simulink model "purePursuitUSCity"  (R2022b)
settings: Solver=VariableStepAuto  StartTime=0.0  StopTime=Ts  RelTol=1e-3
PreLoadFcn:
  | setUpPurePursuitUSCity
model workspace (MAT data in the model file):
  firstWarning = 0
  originalScenarioChecksum = 'F73A6DA3C723D3CA73A6F931B7A52A9C'
values from neighbouring files (symbols this model uses):
  diffcurve = []    [setUpPurePursuitUSCity.m]
  L = data.ActorSpecifications.Length    [setUpPurePursuitUSCity.m]
  ld = 5    [setUpPurePursuitUSCity.m]
  psi_o = refPose(1,3)    [setUpPurePursuitUSCity.m]
  s = size(xRef)    [setUpPurePursuitUSCity.m]
  X_o = refPose(1,1)    [setUpPurePursuitUSCity.m]
  xRef = refPose(:,1)    [setUpPurePursuitUSCity.m]
  Y_o = -refPose(1,2)    [setUpPurePursuitUSCity.m]
  yRef = -refPose(:,2)    [setUpPurePursuitUSCity.m]
undefined symbols (not defined in the file or in its folder): data, deg, rad
libraries: autolibutils x4, autolibshared x3, vehdynlibviscommon x1, aerolibconvert2 x1, simulink_extras x1, drivingscenarioandsensors x1, robotalgslib x1, simulink x1, sim3dlib x1, vdynlib x1
(part 3 of 3)

== system purePursuitUSCity/Powertrain & Driveline/Driveline/FWD ==
  TPowertrain : Inport
  FWD : Gain  Gain=[1;1;0;0]
  TAxles : Outport  VectorParamsAs1DForOutWhenUnconnected=off
  wires:
  FWD/1 -> TAxles/1
  TPowertrain/1 -> FWD/1

== system purePursuitUSCity/Powertrain & Driveline/Driveline/RWD ==
  TPowertrain : Inport
  RWD : Gain  Gain=[0;0;1;1]
  TAxles : Outport  VectorParamsAs1DForOutWhenUnconnected=off
  wires:
  TPowertrain/1 -> RWD/1
  RWD/1 -> TAxles/1

== matlab function purePursuitUSCity/Final Trajectory Bird's-Eye Visualization/MATLAB Function ==
  data: pos input; egoActor output Bus: BusActorsActors; vel input; yaw input; yawRate input
function egoActor = packEgo(pos,vel,yaw,yawRate)
% Pack ego information into a single ego actor bus
%
% Imoprtant note:
% Output is a bus of type BusActorsActors. This is the same bus used by the
% Scenario Reader to output an individual actor. If you change the
% output bus name of Scenario Reader, change the output bus name here
% as well by clicking on 'Edit Data' in the menu above.

egoActor = struct(...
    'ActorID',67,...
    'Position', [pos(1) pos(2) 0], ...
    'Velocity', [vel(1) vel(2) 0], ...
    'Roll', 0, ...
    'Pitch', 0, ...
    'Yaw', yaw, ...
    'AngularVelocity', [0 0 yawRate]);

== matlab function purePursuitUSCity/Optimal Vel/MATLAB Function ==
  data: diffcurve input; y output; speed input; cx input; cy input; refX input; refY input; j output; j input
function [y,j]= fcn(diffcurve,speed,cx,cy,refX,refY,j)

dx = refX- x;
dy = [refY- y];
d= hypot(dx, dy);
[~, ind] = min(d);


if(j==floor(ind/10)) 
    
    if diffcurve(j)>0 && diffcurve(j)<0.5
        %vel(end+1)=30;
        speed=30;
        
    data.ActorSpecifications.Speed=speed;
    y=data.ActorSpecifications.Speed;
    
    elseif diffcurve(j)>=0.5 && diffcurve(j)<1
        %vel(end+1)=20;
        speed=20;
        
    data.ActorSpecifications.Speed=speed;
    y=data.ActorSpecifications.Speed;
    
    elseif diffcurve(j)>=1 && diffcurve(j)<1.5
        %vel(end+1)=10;
        speed=10;
    
    data.ActorSpecifications.Speed=speed;
    y=data.ActorSpecifications.Speed;
    
    elseif diffcurve(j)>=1.5 && diffcurve(j)<2
        %vel(end+1)=5;
        speed=5;
    
    data.ActorSpecifications.Speed=speed;
    y=data.ActorSpecifications.Speed;
    
    else
        %vel(end+1)=3;
        speed=3;
    
    data.ActorSpecifications.Speed=speed;
    y=data.ActorSpecifications.Speed;
    
    end
    j=j+1;
    
end
end
% for i=1:length(diffcurve)-1
%     if diffcurve(i)>0 && diffcurve(i)<0.5
%         %vel(end+1)=30;
%         speed=30;
%     elseif diffcurve(i)>=0.5 && diffcurve(i)<1
%         %vel(end+1)=20;
%         speed=20;
%     elseif diffcurve(i)>=1 && diffcurve(i)<1.5
%         %vel(end+1)=10;
%         speed=10;
%     elseif diffcurve(i)>=1.5 && diffcurve(i)<2
%         %vel(end+1)=5;
%         speed=5;
%     else
%         %vel(end+1)=3;
%         speed=3;
%     end
%     data.ActorSpecifications.Speed=speed;
%     y=data.ActorSpecifications.Speed;
% end
